simulink model "Verification_6DOF_Block"  (R2020a)
settings: Solver=ode4  StartTime=0.0  StopTime=15  FixedStep=0.01  RelTol=1e-3
values from neighbouring files (symbols this model uses):
  m = 15    [RBDsolvertest.m]
libraries: shared6dof x1
settings Model: Creator=mohan  LastModifiedBy=mohan

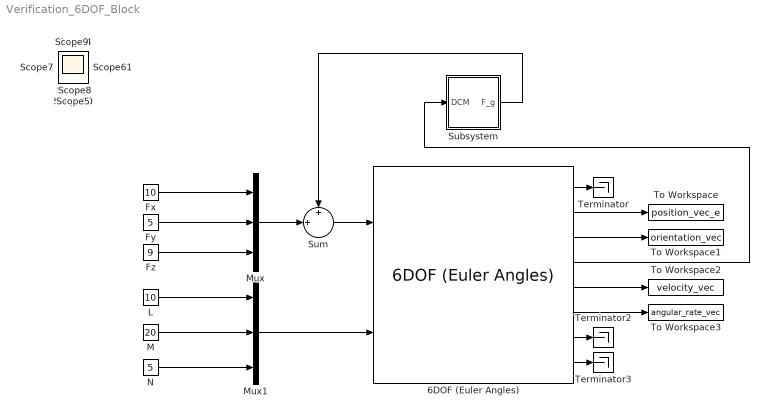
== system Verification_6DOF_Block ==
  6DOF (Euler Angles) : shared6dof/6DOF (Euler Angles)  units=Metric (MKS)  mtype=Fixed  rep=Euler Angles  xme_0=[2 4 7]  Vm_0=[10 2 0]  eul_0=[20 15 30]*pi/180  pm_0=[2 1 0]*pi/180  mass_0=15  mass_e=0.5  mass_f=2.0  inertia=[1 -2 -1 ; -2 5 -3 ; -1 -3 0.1]  inertia_e=eye(3)  inertia_f=2*eye(3)  k_quat=1.0  vre_flag=on  abi_flag=off  aMode=0  xme_statename=''  Vm_statename=''  eul_statename=''  quat_statename=''  pm_statename=''  mass_statename=''
      settings: SourceProductBaseCode=AE,PW,MT,VE,VP
  Fx : Constant  Value=10
  Fy : Constant  Value=5
  Fz : Constant  Value=9
  L : Constant  Value=10
  M : Constant  Value=20
  Mux : Mux  Inputs=3
  Mux1 : Mux  Inputs=3
  N : Constant  Value=5
  Subsystem : Subsystem
  Sum : Sum  Inputs=+|+||
  Terminator : Terminator
  Terminator2 : Terminator
  Terminator3 : Terminator
  To Workspace : ToWorkspace  VariableName=position_vec_e  SaveFormat=Timeseries  SampleTime=-1
  To Workspace1 : ToWorkspace  VariableName=orientation_vec  SaveFormat=Timeseries  SampleTime=-1
  To Workspace2 : ToWorkspace  VariableName=velocity_vec  SaveFormat=Timeseries  SampleTime=-1
  To Workspace3 : ToWorkspace  VariableName=angular_rate_vec  SaveFormat=Timeseries  SampleTime=-1
  Scope{,1..11} (12 alike) : Scope
  wires:
  Fx/1 -> Mux/1
  Fy/1 -> Mux/2
  Fz/1 -> Mux/3
  L/1 -> Mux1/1
  M/1 -> Mux1/2
  N/1 -> Mux1/3
  6DOF (Euler Angles)/5 -> To Workspace2/1
  6DOF (Euler Angles)/1 -> Terminator/1
  6DOF (Euler Angles)/7 -> Terminator2/1
  6DOF (Euler Angles)/8 -> Terminator3/1
  6DOF (Euler Angles)/2 -> To Workspace/1
  6DOF (Euler Angles)/6 -> To Workspace3/1
  Mux1/1 -> 6DOF (Euler Angles)/2
  6DOF (Euler Angles)/3 -> To Workspace1/1
  Mux/1 -> Sum/2
  Subsystem/1(F_g) -> Sum/1
  Sum/1 -> 6DOF (Euler Angles)/1
  6DOF (Euler Angles)/4 -> Subsystem/1(DCM)

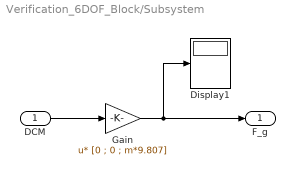
== system Verification_6DOF_Block/Subsystem ==
  DCM : Inport
  Display1 : Display
  Gain : Gain  Gain=[0 ; 0 ; m*9.807]  Multiplication=Matrix(u*K)
  F_g : Outport
  wires:
  Gain/1 -> F_g/1, Display1/1
  DCM/1 -> Gain/1
